simulink model "task3"  (R2022b)
settings: Solver=FixedStepAuto  StartTime=0.0  StopTime=10.0  RelTol=1e-8
settings Model: Creator=anton  LastModifiedBy=anton
settings DataIOCC: ExternalInput=data  LoadExternalInput=on

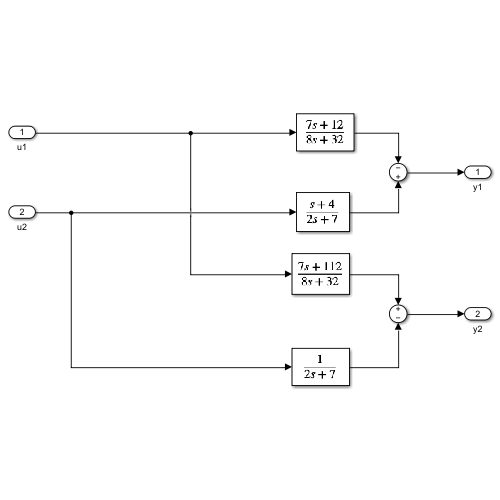
[thumbnail: Simulink's stored preview of the top-level diagram]
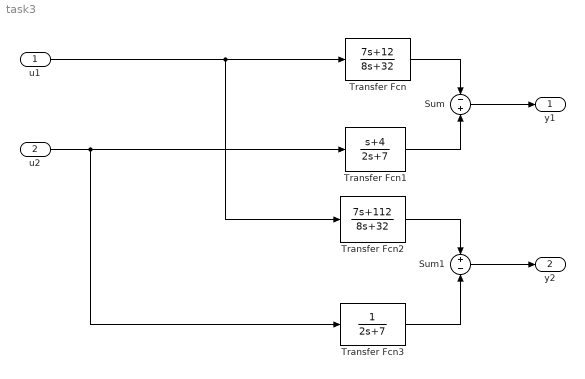
== system task3 ==
  u1 : Inport  PortDimensions=1
  u2 : Inport  Port=2  PortDimensions=1
  Sum : Sum  Inputs=-+
  Sum1 : Sum  Inputs=+-
  Transfer Fcn : TransferFcn  Numerator=[7 12]  Denominator=[8 32]
  Transfer Fcn1 : TransferFcn  Numerator=[1 4]  Denominator=[2 7]
  Transfer Fcn2 : TransferFcn  Numerator=[7 112]  Denominator=[8 32]
  Transfer Fcn3 : TransferFcn  Denominator=[2 7]
  y1 : Outport
  y2 : Outport  Port=2
  wires:
  Transfer Fcn/1 -> Sum/1
  Transfer Fcn1/1 -> Sum/2
  Transfer Fcn3/1 -> Sum1/2
  Transfer Fcn2/1 -> Sum1/1
  u2/1 -> Transfer Fcn3/1, Transfer Fcn1/1
  u1/1 -> Transfer Fcn2/1, Transfer Fcn/1
  Sum1/1 -> y2/1
  Sum/1 -> y1/1
